simulink subsystem "Euler_Eqns_Vector"  (R2022b)
settings: Solver=VariableStepAuto  StartTime=0.0  StopTime=10.0  RelTol=1e-3
undefined symbols (not defined in the file or in its folder): I, w0
libraries: matrix_library x1
settings Model: Creator=robertopistonenascone  LastModifiedBy=robertopistonenascone

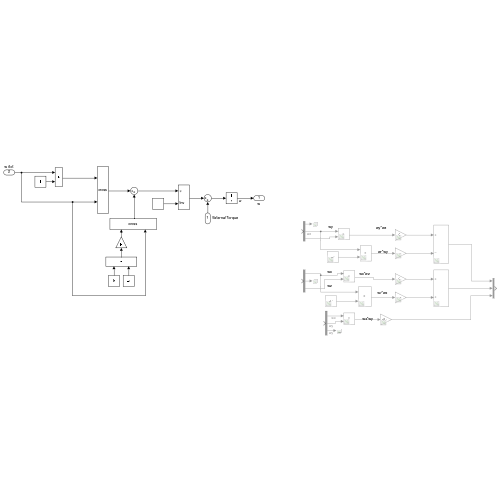
[thumbnail: Simulink's stored preview of the top-level diagram]
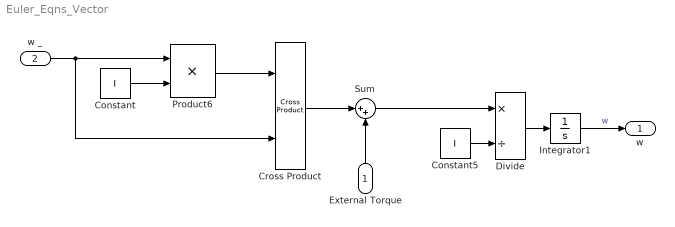
== system Euler_Eqns_Vector ==
  External Torque : Inport
  w _ : Inport  Port=2
  Constant : Constant  Value=I
  Constant5 : Constant  Value=I
  Cross Product : matrix_library/Cross Product
  Divide : Product  Inputs=*/
  Integrator1 : Integrator  InitialCondition=w0
  Product6 : Product
  Sum : Sum  Inputs=|++
  w : Outport
  wires:
  Cross Product/1 -> Sum/1
  Product6/1 -> Cross Product/1
  Divide/1 -> Integrator1/1
  w _/1 -> Product6/1, Cross Product/2
  Constant/1 -> Product6/2
  Constant5/1 -> Divide/2
  External Torque/1 -> Sum/2
  Integrator1/1 -> w/1  "w"
  Sum/1 -> Divide/1
